simulink model "external_memory_test"  (R2020b)
settings: Solver=FixedStepDiscrete  StartTime=0.0  StopTime=80  RelTol=1e-3
InitFcn:
  | Feature_Width = 64;
  | Feature_Height = 64;
  | Weight_Width = 3;
  | Weight_Height = 3;
  | external_memory_test_init;
values from neighbouring files (symbols this model uses):
  Burst_Length = Feature_Weight_Length    [external_memory_test_init.m]
  byPass = 1    [external_memory_test_init.m]
  Conv_Padding = 0    [external_memory_test_init.m]
  Conv_Stride = 1    [external_memory_test_init.m]
  DDR_Depth = Weight_Length + Feature_Length + outFeature_Length    [external_memory_test_init.m]
  ddrInitData = single((rand(1,DDR_Depth)))    [external_memory_test_init.m]
  Duty_Cycle = 0.5    [external_memory_test_init.m]
  Feature_Area = Feature_Width * Feature_Height    [external_memory_test_init.m]
  Feature_Length = Phase_In * Feature_Area    [external_memory_test_init.m]
  inChannel = 3    [external_memory_test_init.m]
  outChannel = 2    [external_memory_test_init.m]
  outFeature_Length = outFeature_Width * outFeature_Height * Phase_Out    [external_memory_test_init.m]
  Pool_Stride = 2    [external_memory_test_init.m]
  Pool_Width = 2    [external_memory_test_init.m]
  Tc = 1    [external_memory_test_init.m]
  Ti = 1    [external_memory_test_init.m]
  To = 1    [external_memory_test_init.m]
  Tr = 1    [external_memory_test_init.m]
  Weight_Length = Phase_In * Weight_Area * Phase_Out    [external_memory_test_init.m]
undefined symbols (not defined in the file or in its folder): Conv_Step, Pool_Step, sigbuilder_block
libraries: hdlsllib x85, simulink x44, visionhdlutilities x16
(part 5 of 6)

== system external_memory_test/DUT/2DConvPE V1.3/Address Logic/  ==
  In1 : Inport
  In2 : Inport  Port=2
  Constant1 : Constant  Value=0  OutDataTypeStr=uint32
  Constant2 : Constant  Value=0  OutDataTypeStr=uint32
  Logical Operator3 : Logic  Operator=NOT  AllPortsSameDT=off  OutDataTypeStr=boolean
  Switch : Switch  Criteria=u2 ~= 0
  Switch1 : Switch  Criteria=u2 ~= 0
  addr_bit_sel1 : hdlsllib/Logic and Bit Operations/Bit Slice  lidx=12  ridx=0
  addr_bit_sel2 : hdlsllib/Logic and Bit Operations/Bit Slice  lidx=12  ridx=0
  W : Outport
  R : Outport  Port=2
  wires:
  In2/1 -> Switch/2, Logical Operator3/1
  Constant1/1 -> Switch/1
  Switch1/1 -> addr_bit_sel1/1
  In1/1 -> Switch1/3, Switch/3
  Logical Operator3/1 -> Switch1/2
  Constant2/1 -> Switch1/1
  Switch/1 -> addr_bit_sel2/1
  addr_bit_sel1/1 -> W/1  "vec_wr_addr"
  addr_bit_sel2/1 -> R/1  "vec_wr_addr"

== system external_memory_test/DUT/2DConvPE V1.3/LIne Buffer/Line Buffer ==
  Stream_In : Inport
  Stream_Valid : Inport  Port=2
  Feature_Area : Inport  Port=3
  Feature_Width : Inport  Port=4
  CtrlGen : Subsystem
  Line Buffer : visionhdlutilities/Line Buffer  NeighborhoodSize=[3 1]  PaddingMethod=Constant  PaddingValue=0  LineBufferSize=128  SimulateUsing=Code generation
      settings: SourceProductBaseCode=VT
  pixel : Outport
  ctrl : Outport  Port=2
  shftEnable : Outport  Port=3
  wires:
  Feature_Area/1 -> CtrlGen/3(Feature_Area)
  Line Buffer/2 -> ctrl/1
  CtrlGen/1(StreamOut) -> Line Buffer/1
  Feature_Width/1 -> CtrlGen/4(Feature_Width)
  Stream_In/1 -> CtrlGen/1(Stream_In)
  CtrlGen/2(Ctrl) -> Line Buffer/2
  Stream_Valid/1 -> CtrlGen/2(Stream_Valid)
  Line Buffer/3 -> shftEnable/1
  Line Buffer/1 -> pixel/1

== system external_memory_test/DUT/2DConvPE V1.3/LIne Buffer/OutValidGen ==
  In1 : Inport
  Weight_Width : Inport  Port=2
  Feature_Height : Inport  Port=3
  Compare To Constant : simulink/Logic and Bit Operations/Compare To Constant  relop=>  const=0  OutDataTypeStr=boolean
  Constant : Constant  OutDataTypeStr=uint32  SampleTime=-1
  Delay2 : Delay  DelayLength=1
  Logical Operator1 : Logic  Operator=NOT  AllPortsSameDT=off  OutDataTypeStr=boolean
  Logical Operator2 : Logic  Operator=OR  AllPortsSameDT=off  OutDataTypeStr=boolean
  Logical Operator3 : Logic  Inputs=4  AllPortsSameDT=off  OutDataTypeStr=boolean
  Logical Operator4 : Logic  Operator=NOT  AllPortsSameDT=off  OutDataTypeStr=boolean
  Logical Operator5 : Logic  Operator=OR  AllPortsSameDT=off  OutDataTypeStr=boolean
  Logical Operator6 : Logic  Operator=NOT  Inputs=3  AllPortsSameDT=off  OutDataTypeStr=boolean
  Minus1 : Sum  Inputs=+--
  Minus2 : Sum  Inputs=+-
  NumRow_Counter : hdlsllib/Sources/HDL Counter  CountType=Free running  CountInit=0  CountStep=1  CountMax=2^15  CountFromType=Initial value  CountFrom=0  CountResetPort=on  CountLoadPort=off  CountEnbPort=on  CountDirPort=off  CountDataType=Unsigned  CountWordLen=32  CountFracLen=0  CountSampTime=1
  Pixel Control Bus Selector : BusSelector  OutputSignals=hStart,hEnd,vStart,vEnd,valid
  Relational Operator1 : RelationalOperator  Operator=<  OutDataTypeStr=boolean  RndMeth=Nearest
  Relational Operator2 : RelationalOperator  Operator=<=  OutDataTypeStr=boolean  RndMeth=Nearest
  Row_Counter : hdlsllib/Sources/HDL Counter  CountType=Free running  CountInit=0  CountStep=1  CountMax=2^15  CountFromType=Initial value  CountFrom=0  CountResetPort=on  CountLoadPort=off  CountEnbPort=on  CountDirPort=off  CountDataType=Unsigned  CountWordLen=32  CountFracLen=0  CountSampTime=1
  Terminator1 : Terminator
  valid : Outport
  wires:
  Compare To Constant/1 -> Logical Operator3/2
  NumRow_Counter/1 -> Relational Operator2/2, Compare To Constant/1
  Pixel Control Bus Selector/1 -> NumRow_Counter/2, Logical Operator2/1  "<hStart>"
  Minus2/1 -> Relational Operator2/1
  Relational Operator1/1 -> Logical Operator4/1
  Logical Operator1/1 -> Logical Operator2/2
  Pixel Control Bus Selector/3 -> Logical Operator5/1  "<vStart>"
  Feature_Height/1 -> Minus2/1
  Minus1/1 -> Relational Operator1/2
  Row_Counter/1 -> Relational Operator1/1
  Pixel Control Bus Selector/5 -> Logical Operator1/1, Row_Counter/2, Logical Operator3/3  "<valid>"
  Weight_Width/1 -> Minus1/1
  Pixel Control Bus Selector/2 -> Terminator1/1  "<hEnd>"
  Delay2/1 -> Pixel Control Bus Selector/1
  Constant/1 -> Minus1/3, Minus1/2, Minus2/2
  Logical Operator6/1 -> Logical Operator3/1
  Logical Operator5/1 -> NumRow_Counter/1
  Pixel Control Bus Selector/4 -> Logical Operator5/2  "<vEnd>"
  Relational Operator2/1 -> Logical Operator6/1
  Logical Operator2/1 -> Row_Counter/1
  Logical Operator4/1 -> Logical Operator3/4
  Logical Operator3/1 -> valid/1
  In1/1 -> Delay2/1

== system external_memory_test/DUT/2DConvPE V1.3/MaxPooling/Comparator ==
  In1 : Inport
  In2 : Inport  Port=2
  In3 : Inport  Port=3
  In4 : Inport  Port=4
  Valid : Inport  Port=5
  Delay{,1..4} (5 alike) : Delay  DelayLength=1
  Relational Operator : RelationalOperator  Operator=>  OutDataTypeStr=boolean  RndMeth=Nearest
  Relational Operator1 : RelationalOperator  Operator=>  OutDataTypeStr=boolean  RndMeth=Nearest
  Relational Operator2 : RelationalOperator  Operator=>  OutDataTypeStr=boolean  RndMeth=Nearest
  Switch : Switch  Criteria=u2 > Threshold
  Switch1 : Switch  Criteria=u2 > Threshold
  Switch2 : Switch  Criteria=u2 > Threshold
  Out1 : Outport
  outvalid : Outport  Port=2
  wires:
  Switch1/1 -> Relational Operator2/2, Switch2/3
  Switch/1 -> Switch2/1, Relational Operator2/1
  Delay/1 -> Switch/1, Relational Operator/1
  Relational Operator/1 -> Switch/2
  Relational Operator1/1 -> Switch1/2
  In2/1 -> Delay1/1
  In3/1 -> Delay2/1
  Relational Operator2/1 -> Switch2/2
  In4/1 -> Delay3/1
  Switch2/1 -> Out1/1
  Valid/1 -> Delay4/1
  Delay1/1 -> Relational Operator/2, Switch/3
  Delay2/1 -> Switch1/1, Relational Operator1/1
  In1/1 -> Delay/1
  Delay3/1 -> Relational Operator1/2, Switch1/3
  Delay4/1 -> outvalid/1

== system external_memory_test/DUT/2DConvPE V1.3/MaxPooling/Line Buffer1 ==
  Stream_In : Inport
  Stream_Valid : Inport  Port=2
  Feature_Area : Inport  Port=3
  Feature_Width : Inport  Port=4
  CtrlGen : Subsystem
  Line Buffer : visionhdlutilities/Line Buffer  NeighborhoodSize=[2 1]  PaddingMethod=Constant  PaddingValue=0  LineBufferSize=128  SimulateUsing=Code generation
      settings: SourceProductBaseCode=VT
  pixel : Outport
  ctrl : Outport  Port=2
  shftEnable : Outport  Port=3
  wires:
  Feature_Area/1 -> CtrlGen/3(Feature_Area)
  Line Buffer/2 -> ctrl/1
  CtrlGen/1(StreamOut) -> Line Buffer/1
  Feature_Width/1 -> CtrlGen/4(Feature_Width)
  Stream_In/1 -> CtrlGen/1(Stream_In)
  CtrlGen/2(Ctrl) -> Line Buffer/2
  Stream_Valid/1 -> CtrlGen/2(Stream_Valid)
  Line Buffer/3 -> shftEnable/1
  Line Buffer/1 -> pixel/1

== system external_memory_test/DUT/2DConvPE V1.3/MaxPooling/OutValidGen ==
  ctrl : Inport
  Window_Width : Inport  Port=2
  Feature_Height : Inport  Port=3
  Compare To Constant : simulink/Logic and Bit Operations/Compare To Constant  Commented=on  relop=>  const=0  OutDataTypeStr=boolean
  Constant : Constant  OutDataTypeStr=uint32  SampleTime=-1
  Delay36 : Delay  DelayLength=1
  Logical Operator1 : Logic  Operator=NOT  AllPortsSameDT=off  OutDataTypeStr=boolean
  Logical Operator3 : Logic  Inputs=3  AllPortsSameDT=off  OutDataTypeStr=boolean
  Logical Operator4 : Logic  Operator=NOT  AllPortsSameDT=off  OutDataTypeStr=boolean
  Logical Operator5 : Logic  Operator=OR  AllPortsSameDT=off  OutDataTypeStr=boolean
  Logical Operator6 : Logic  Operator=NOT  Inputs=3  AllPortsSameDT=off  OutDataTypeStr=boolean
  Minus1 : Sum  Inputs=+-
  Minus2 : Sum  Inputs=+-
  NumRow_Counter : hdlsllib/Sources/HDL Counter  CountType=Free running  CountInit=0  CountStep=1  CountMax=2^15  CountFromType=Initial value  CountFrom=0  CountResetPort=on  CountLoadPort=off  CountEnbPort=on  CountDirPort=off  CountDataType=Unsigned  CountWordLen=32  CountFracLen=0  CountSampTime=1
  Pixel Control Bus Selector : BusSelector  OutputSignals=hStart,hEnd,vStart,vEnd,valid
  Relational Operator1 : RelationalOperator  Operator=<  OutDataTypeStr=boolean  RndMeth=Nearest
  Relational Operator2 : RelationalOperator  Operator=<=  OutDataTypeStr=boolean  RndMeth=Nearest
  Row_Counter : hdlsllib/Sources/HDL Counter  CountType=Free running  CountInit=0  CountStep=1  CountMax=2^15  CountFromType=Initial value  CountFrom=0  CountResetPort=on  CountLoadPort=off  CountEnbPort=on  CountDirPort=off  CountDataType=Unsigned  CountWordLen=32  CountFracLen=0  CountSampTime=1
  Terminator1 : Terminator
  Out1 : Outport
  wires:
  NumRow_Counter/1 -> Relational Operator2/2, Compare To Constant/1
  Pixel Control Bus Selector/1 -> NumRow_Counter/2  "<hStart>"
  Minus2/1 -> Relational Operator2/1
  Relational Operator1/1 -> Logical Operator4/1
  Pixel Control Bus Selector/3 -> Logical Operator5/1  "<vStart>"
  Feature_Height/1 -> Minus2/1
  Minus1/1 -> Relational Operator1/2
  Row_Counter/1 -> Relational Operator1/1
  Pixel Control Bus Selector/5 -> Row_Counter/2, Logical Operator1/1, Logical Operator3/2  "<valid>"
  Window_Width/1 -> Minus1/1
  Pixel Control Bus Selector/2 -> Terminator1/1  "<hEnd>"
  Delay36/1 -> Pixel Control Bus Selector/1
  Constant/1 -> Minus1/2, Minus2/2
  Logical Operator6/1 -> Logical Operator3/1
  Logical Operator5/1 -> NumRow_Counter/1
  Pixel Control Bus Selector/4 -> Logical Operator5/2  "<vEnd>"
  Relational Operator2/1 -> Logical Operator6/1
  Logical Operator1/1 -> Row_Counter/1
  Logical Operator4/1 -> Logical Operator3/3
  Logical Operator3/1 -> Out1/1
  ctrl/1 -> Delay36/1

== system external_memory_test/DUT/2DConvPE V1.3/MaxPooling/window Selector ==
  pixel : Inport
  valid : Inport  Port=2
  step : Inport  Port=3
  Add : Sum  Inputs=+-
  Compare To Zero : simulink/Logic and Bit Operations/Compare To Zero  relop===  OutDataTypeStr=boolean
  Constant : Constant  OutDataTypeStr=uint32
  Delay : Delay
  Delay1 : Delay  DelayLength=1
  Delay36 : Delay  DelayLength=1
  Logical Operator : Logic  Operator=NOT  AllPortsSameDT=off  OutDataTypeStr=boolean
  Logical Operator1 : Logic  Operator=OR  AllPortsSameDT=off  OutDataTypeStr=boolean
  Logical Operator2 : Logic  AllPortsSameDT=off  OutDataTypeStr=boolean
  Relational Operator : RelationalOperator  OutDataTypeStr=boolean  RndMeth=Nearest
  Selector1 : Selector  InputPortWidth=2  IndexOptions=Index vector (dialog)  Indices=[1]  OutputSizes=1
  Selector2 : Selector  InputPortWidth=2  IndexOptions=Index vector (dialog)  Indices=[2]  OutputSizes=1
  Selector3 : Selector  InputPortWidth=2  IndexOptions=Index vector (dialog)  Indices=[1]  OutputSizes=1
  Selector4 : Selector  InputPortWidth=2  IndexOptions=Index vector (dialog)  Indices=[2]  OutputSizes=1
  Step Counter : hdlsllib/Sources/HDL Counter  CountType=Free running  CountInit=0  CountStep=1  CountMax=2^15  CountFromType=Initial value  CountFrom=0  CountResetPort=on  CountLoadPort=off  CountEnbPort=on  CountDirPort=off  CountDataType=Unsigned  CountWordLen=32  CountFracLen=0  CountSampTime=1
  Out1 : Outport
  Out2 : Outport  Port=2
  Out3 : Outport  Port=3
  Out4 : Outport  Port=4
  Valid : Outport  Port=5
  wires:
  Selector2/1 -> Out2/1
  Delay/1 -> Selector4/1, Selector3/1
  Selector3/1 -> Out3/1
  Selector1/1 -> Out1/1
  Selector4/1 -> Out4/1
  pixel/1 -> Delay36/1, Delay/1
  Step Counter/1 -> Compare To Zero/1, Relational Operator/1
  Delay1/1 -> Logical Operator2/2, Step Counter/2, Logical Operator/1
  Logical Operator/1 -> Logical Operator1/2
  step/1 -> Add/1
  Constant/1 -> Add/2
  Add/1 -> Relational Operator/2
  Relational Operator/1 -> Logical Operator1/1
  Logical Operator1/1 -> Step Counter/1
  Compare To Zero/1 -> Logical Operator2/1
  Logical Operator2/1 -> Valid/1
  Delay36/1 -> Selector2/1, Selector1/1
  valid/1 -> Delay1/1

== system external_memory_test/DUT/Input Buffer/OutAddressLogic/FeatureAddressOut ==
  note: FeatureDelay May Correlated to Line Buffer Window
  Feature_Length : Inport
  Out_Enable : Inport  Port=2
  Feature_Width : Inport  Port=3
  outChannel : Inport  Port=4
  Feature_Height : Inport  Port=5
  " FeatureDelay" : Constant  OutDataTypeStr=uint32  SampleTime=-1
  Add{1..2,4,6} (4 alike) : Sum  Inputs=+-
  Add3 : Sum
  Add5 : Sum
  Constant1 : Constant  OutDataTypeStr=uint32  SampleTime=-1
  Feature_Length_Counter : hdlsllib/Sources/HDL Counter  CountType=Free running  CountInit=0  CountStep=1  CountMax=2^15  CountFromType=Initial value  CountFrom=0  CountResetPort=on  CountLoadPort=off  CountEnbPort=on  CountDirPort=off  CountDataType=Unsigned  CountWordLen=32  CountFracLen=0  CountSampTime=1
  Iteration_Counter : hdlsllib/Sources/HDL Counter  CountType=Free running  CountInit=0  CountStep=1  CountMax=2^15  CountFromType=Initial value  CountFrom=0  CountResetPort=on  CountLoadPort=off  CountEnbPort=on  CountDirPort=off  CountDataType=Unsigned  CountWordLen=32  CountFracLen=0  CountSampTime=1
  Logical Operator{,2,4..5} (4 alike) : Logic  Operator=NOT  AllPortsSameDT=off  OutDataTypeStr=boolean
  Logical Operator1 : Logic  Inputs=3  AllPortsSameDT=off  OutDataTypeStr=boolean
  Logical Operator3 : Logic  AllPortsSameDT=off  OutDataTypeStr=boolean
  Logical Operator6 : Logic  Operator=OR  AllPortsSameDT=off  OutDataTypeStr=boolean
  Relational Operator{1..6} (6 alike) : RelationalOperator  Operator=>  OutDataTypeStr=boolean  RndMeth=Simplest
  Row+Delay_Counter : hdlsllib/Sources/HDL Counter  CountType=Free running  CountInit=0  CountStep=1  CountMax=2^15  CountFromType=Initial value  CountFrom=0  CountResetPort=on  CountLoadPort=off  CountEnbPort=on  CountDirPort=off  CountDataType=Unsigned  CountWordLen=32  CountFracLen=0  CountSampTime=1
  RowDelay : Constant  OutDataTypeStr=uint32  SampleTime=-1
  Row_Counter : hdlsllib/Sources/HDL Counter  CountType=Free running  CountInit=0  CountStep=1  CountMax=2^15  CountFromType=Initial value  CountFrom=0  CountResetPort=on  CountLoadPort=off  CountEnbPort=on  CountDirPort=off  CountDataType=Unsigned  CountWordLen=32  CountFracLen=0  CountSampTime=1
  count : Outport
  Out2 : Outport  Port=2
  PhaseOut_Count : Outport  Port=3
  wires:
  RowDelay/1 -> Add3/1
  Out_Enable/1 -> Logical Operator3/2, Logical Operator4/1
  Row+Delay_Counter/1 -> Relational Operator2/1, Relational Operator1/1
  Add4/1 -> Relational Operator4/2
  Constant1/1 -> Add6/2, Add2/2, Add4/2, Add1/2
  Relational Operator3/1 -> Feature_Length_Counter/1, Iteration_Counter/2
  Logical Operator1/1 -> Out2/1, Feature_Length_Counter/2
  Iteration_Counter/1 -> Relational Operator4/1, PhaseOut_Count/1
  Relational Operator4/1 -> Logical Operator2/1
  Relational Operator2/1 -> Logical Operator/1
  Logical Operator3/1 -> Row+Delay_Counter/2, Logical Operator1/1
  Add1/1 -> Relational Operator3/2
  Add3/1 -> Relational Operator1/2
  Relational Operator1/1 -> Logical Operator6/1, Row_Counter/2
  Logical Operator4/1 -> Iteration_Counter/1
  Add2/1 -> Relational Operator2/2, Add3/2
  Logical Operator/1 -> Logical Operator1/2
  Feature_Length_Counter/1 -> count/1, Relational Operator3/1
  Logical Operator2/1 -> Logical Operator3/1
  Feature_Width/1 -> Add2/1
  Feature_Length/1 -> Add1/1
  outChannel/1 -> Add4/1
  Add5/1 -> Relational Operator5/2
  Row_Counter/1 -> Relational Operator5/1, Relational Operator6/1
  Feature_Height/1 -> Add5/2, Add6/1
  " FeatureDelay"/1 -> Add5/1
  Relational Operator5/1 -> Row_Counter/1, Logical Operator6/2
  Add6/1 -> Relational Operator6/2
  Relational Operator6/1 -> Logical Operator5/1
  Logical Operator5/1 -> Logical Operator1/3
  Logical Operator6/1 -> Row+Delay_Counter/1

== system external_memory_test/DUT/Input Buffer/OutAddressLogic/Subsystem ==
  In1 : Inport
  Feature_Area : Inport  Port=2
  Weight_Length : Inport  Port=3
  Weight_Area : Inport  Port=4
  Add1 : Sum  Inputs=+-
  Add2 : Sum  Inputs=+-
  Add3 : Sum  Inputs=+-
  Constant1 : Constant  OutDataTypeStr=uint32  SampleTime=-1
  Feature_Area_Count : hdlsllib/Sources/HDL Counter  CountType=Free running  CountInit=0  CountStep=1  CountMax=2^15  CountFromType=Initial value  CountFrom=0  CountResetPort=on  CountLoadPort=off  CountEnbPort=on  CountDirPort=off  CountDataType=Unsigned  CountWordLen=32  CountFracLen=0  CountSampTime=1
  Logical Operator1 : Logic  Operator=NOT  AllPortsSameDT=off  OutDataTypeStr=boolean
  Logical Operator2 : Logic  Operator=NOT  AllPortsSameDT=off  OutDataTypeStr=boolean
  Logical Operator3 : Logic  AllPortsSameDT=off  OutDataTypeStr=boolean
  Relational Operator2 : RelationalOperator  Operator=>  OutDataTypeStr=boolean  RndMeth=Simplest
  Relational Operator3 : RelationalOperator  Operator=>  OutDataTypeStr=boolean  RndMeth=Simplest
  Relational Operator4 : RelationalOperator  Operator=<=  OutDataTypeStr=boolean  RndMeth=Simplest
  Weight_Length_Count : hdlsllib/Sources/HDL Counter  CountType=Free running  CountInit=0  CountStep=1  CountMax=2^15  CountFromType=Initial value  CountFrom=0  CountResetPort=on  CountLoadPort=off  CountEnbPort=on  CountDirPort=off  CountDataType=Unsigned  CountWordLen=32  CountFracLen=0  CountSampTime=1
  weight_ram_rd_addr : Outport
  valid : Outport  Port=2
  wires:
  Relational Operator4/1 -> Logical Operator3/2
  Weight_Length/1 -> Add1/1
  Feature_Area/1 -> Add2/1
  Constant1/1 -> Add3/2, Add1/2, Add2/2
  Weight_Length_Count/1 -> weight_ram_rd_addr/1, Relational Operator2/2
  Relational Operator2/1 -> Logical Operator1/1
  Logical Operator3/1 -> valid/1, Weight_Length_Count/2
  Feature_Area_Count/1 -> Relational Operator4/1, Relational Operator3/2
  In1/1 -> Logical Operator3/1, Feature_Area_Count/2
  Add2/1 -> Relational Operator3/1
  Add3/1 -> Relational Operator4/2
  Add1/1 -> Relational Operator2/1
  Logical Operator2/1 -> Feature_Area_Count/1
  Relational Operator3/1 -> Logical Operator2/1
  Logical Operator1/1 -> Weight_Length_Count/1
  Weight_Area/1 -> Add3/1

== system external_memory_test/DUT/Input Buffer/Subsystem1/Subsystem ==
  In1 : Inport
  Bus Selector : BusSelector  OutputSignals=signal1,signal2,signal3,signal4,signal5,signal6,signal7,signal8,signal9,signal10,signal11,signal12,signal13,signal14,signal15
  Weight_Length : Outport
  Weight_Area : Outport  Port=2
  Weight_Width : Outport  Port=3
  Weight_Height : Outport  Port=4
  Feature_Length : Outport  Port=5
  Feature_Area : Outport  Port=6
  Feature_Width : Outport  Port=7
  Feature_Height : Outport  Port=8
  outFeature_Length : Outport  Port=9
  outFeature_Area : Outport  Port=10
  outFeature_Width : Outport  Port=11
  outFeature_Height : Outport  Port=12
  Conv_Step : Outport  Port=13
  inChannel : Outport  Port=14
  outChannel : Outport  Port=15
  wires:
  In1/1 -> Bus Selector/1
  Bus Selector/1 -> Weight_Length/1  "<signal1>"
  Bus Selector/2 -> Weight_Area/1  "<signal2>"
  Bus Selector/3 -> Weight_Width/1  "<signal3>"
  Bus Selector/4 -> Weight_Height/1  "<signal4>"
  Bus Selector/5 -> Feature_Length/1  "<signal5>"
  Bus Selector/6 -> Feature_Area/1  "<signal6>"
  Bus Selector/7 -> Feature_Width/1  "<signal7>"
  Bus Selector/8 -> Feature_Height/1  "<signal8>"
  Bus Selector/9 -> outFeature_Length/1  "<signal9>"
  Bus Selector/10 -> outFeature_Area/1  "<signal10>"
  Bus Selector/11 -> outFeature_Width/1  "<signal11>"
  Bus Selector/12 -> outFeature_Height/1  "<signal12>"
  Bus Selector/13 -> Conv_Step/1  "<signal13>"
  Bus Selector/14 -> inChannel/1  "<signal14>"
  Bus Selector/15 -> outChannel/1  "<signal15>"

== system external_memory_test/DDR/wrLogic/Wr_control/AckGen/edgeDet ==
  ackIn : Inport
  " ackIn==1" : simulink/Logic and Bit Operations/Compare To Constant  relop===  const=1  OutDataTypeStr=boolean
  ackIn Posedge Detect : Logic  IconShape=distinctive  AllPortsSameDT=off  OutDataTypeStr=boolean
  ackIn_d1 : Delay  DelayLength=1
  ackIn_d1==0 : simulink/Logic and Bit Operations/Compare To Constant  relop===  const=0  OutDataTypeStr=boolean
  ackOut : Outport  VectorParamsAs1DForOutWhenUnconnected=off
  wires:
  " ackIn==1"/1 -> ackIn Posedge Detect/2
  ackIn_d1==0/1 -> ackIn Posedge Detect/1
  ackIn Posedge Detect/1 -> ackOut/1
  ackIn_d1/1 -> ackIn_d1==0/1
  ackIn/1 -> " ackIn==1"/1, ackIn_d1/1

== system external_memory_test/DUT/2DConvPE V1.0/LIne Buffer/Line Buffer/CtrlGen ==
  note: valid
  note: vEnd
  note: vStart
  note: hEnd
  note: hstart
  Stream_In : Inport
  Stream_Valid : Inport  Port=2
  Feature_Area : Inport  Port=3
  Feature_Width : Inport  Port=4
  Compare To Zero : simulink/Logic and Bit Operations/Compare To Zero  relop===  OutDataTypeStr=boolean
  Compare To Zero1 : simulink/Logic and Bit Operations/Compare To Zero  relop===  OutDataTypeStr=boolean
  Constant : Constant  OutDataTypeStr=uint32  SampleTime=-1
  Constant1 : Constant  OutDataTypeStr=uint32  SampleTime=-1
  Delay3 : Delay  DelayLength=1
  Delay35 : Delay  DelayLength=1
  Feature Area Counter : hdlsllib/Sources/HDL Counter  CountType=Free running  CountInit=0  CountStep=1  CountMax=2^15  CountFromType=Initial value  CountFrom=0  CountResetPort=on  CountLoadPort=off  CountEnbPort=on  CountDirPort=off  CountDataType=Unsigned  CountWordLen=32  CountFracLen=0  CountSampTime=1
  Feature Row Counter : hdlsllib/Sources/HDL Counter  CountType=Free running  CountInit=0  CountStep=1  CountMax=2^15  CountFromType=Initial value  CountFrom=0  CountResetPort=on  CountLoadPort=off  CountEnbPort=on  CountDirPort=off  CountDataType=Unsigned  CountWordLen=32  CountFracLen=0  CountSampTime=1
  Logical Operator : Logic  Operator=OR  AllPortsSameDT=off  OutDataTypeStr=boolean
  Logical Operator{1..3,5} (4 alike) : Logic  AllPortsSameDT=off  OutDataTypeStr=boolean
  Minus1 : Sum  Inputs=+-
  Minus2 : Sum  Inputs=+-
  Pixel Control Bus Creator : visionhdlutilities/Pixel Control Bus Creator
      settings: SourceProductBaseCode=VT
  Relational Operator1 : RelationalOperator  Operator===  OutDataTypeStr=boolean  RndMeth=Nearest
  Relational Operator2 : RelationalOperator  Operator===  OutDataTypeStr=boolean  RndMeth=Nearest
  Relational Operator3 : RelationalOperator  Operator===  OutDataTypeStr=boolean  RndMeth=Nearest
  StreamOut : Outport
  Ctrl : Outport  Port=2
  wires:
  Minus2/1 -> Relational Operator3/2, Relational Operator2/2
  Feature Row Counter/1 -> Relational Operator2/1, Relational Operator3/1, Compare To Zero/1
  Relational Operator2/1 -> Feature Row Counter/1
  Compare To Zero/1 -> Logical Operator/2
  Relational Operator3/1 -> Logical Operator2/1
  Feature_Area/1 -> Minus1/1
  Constant/1 -> Minus1/2
  Logical Operator/1 -> Logical Operator1/1
  Constant1/1 -> Minus2/2
  Feature_Width/1 -> Minus2/1
  Pixel Control Bus Creator/1 -> Ctrl/1
  Delay3/1 -> Feature Area Counter/2, Feature Row Counter/2, Logical Operator5/2, Logical Operator2/2, Logical Operator1/2, Logical Operator3/2, Pixel Control Bus Creator/5
  Stream_In/1 -> Delay35/1
  Logical Operator1/1 -> Pixel Control Bus Creator/1
  Logical Operator2/1 -> Pixel Control Bus Creator/2
  Logical Operator3/1 -> Pixel Control Bus Creator/4
  Logical Operator5/1 -> Pixel Control Bus Creator/3
  Feature Area Counter/1 -> Compare To Zero1/1, Relational Operator1/1
  Minus1/1 -> Relational Operator1/2
  Relational Operator1/1 -> Feature Area Counter/1, Logical Operator3/1
  Compare To Zero1/1 -> Logical Operator/1, Logical Operator5/1
  Delay35/1 -> StreamOut/1
  Stream_Valid/1 -> Delay3/1

== system external_memory_test/DUT/2DConvPE V1.0/MaxPooling/Line Buffer1/CtrlGen ==
  note: valid
  note: vEnd
  note: vStart
  note: hEnd
  note: hstart
  Stream_In : Inport
  Stream_Valid : Inport  Port=2
  Feature_Area : Inport  Port=3
  Feature_Width : Inport  Port=4
  Compare To Zero : simulink/Logic and Bit Operations/Compare To Zero  relop===  OutDataTypeStr=boolean
  Compare To Zero1 : simulink/Logic and Bit Operations/Compare To Zero  relop===  OutDataTypeStr=boolean
  Constant : Constant  OutDataTypeStr=uint32  SampleTime=-1
  Constant1 : Constant  OutDataTypeStr=uint32  SampleTime=-1
  Delay1 : Delay  DelayLength=1
  Delay36 : Delay  DelayLength=1
  Feature Area Counter : hdlsllib/Sources/HDL Counter  CountType=Free running  CountInit=0  CountStep=1  CountMax=2^15  CountFromType=Initial value  CountFrom=0  CountResetPort=on  CountLoadPort=off  CountEnbPort=on  CountDirPort=off  CountDataType=Unsigned  CountWordLen=32  CountFracLen=0  CountSampTime=1
  Feature Row Counter : hdlsllib/Sources/HDL Counter  CountType=Free running  CountInit=0  CountStep=1  CountMax=2^15  CountFromType=Initial value  CountFrom=0  CountResetPort=on  CountLoadPort=off  CountEnbPort=on  CountDirPort=off  CountDataType=Unsigned  CountWordLen=32  CountFracLen=0  CountSampTime=1
  Logical Operator : Logic  Operator=OR  AllPortsSameDT=off  OutDataTypeStr=boolean
  Logical Operator{1..3,5} (4 alike) : Logic  AllPortsSameDT=off  OutDataTypeStr=boolean
  Minus1 : Sum  Inputs=+-
  Minus2 : Sum  Inputs=+-
  Pixel Control Bus Creator : visionhdlutilities/Pixel Control Bus Creator
      settings: SourceProductBaseCode=VT
  Relational Operator1 : RelationalOperator  Operator===  OutDataTypeStr=boolean  RndMeth=Nearest
  Relational Operator2 : RelationalOperator  Operator===  OutDataTypeStr=boolean  RndMeth=Nearest
  Relational Operator3 : RelationalOperator  Operator===  OutDataTypeStr=boolean  RndMeth=Nearest
  StreamOut : Outport
  Ctrl : Outport  Port=2
  wires:
  Minus2/1 -> Relational Operator3/2, Relational Operator2/2
  Feature Row Counter/1 -> Relational Operator2/1, Relational Operator3/1, Compare To Zero/1
  Relational Operator2/1 -> Feature Row Counter/1
  Compare To Zero/1 -> Logical Operator/2
  Relational Operator3/1 -> Logical Operator2/1
  Feature_Area/1 -> Minus1/1
  Constant/1 -> Minus1/2
  Logical Operator/1 -> Logical Operator1/1
  Constant1/1 -> Minus2/2
  Feature_Width/1 -> Minus2/1
  Pixel Control Bus Creator/1 -> Ctrl/1
  Delay1/1 -> Feature Area Counter/2, Feature Row Counter/2, Logical Operator5/2, Logical Operator2/2, Logical Operator1/2, Logical Operator3/2, Pixel Control Bus Creator/5
  Delay36/1 -> StreamOut/1
  Logical Operator1/1 -> Pixel Control Bus Creator/1
  Logical Operator2/1 -> Pixel Control Bus Creator/2
  Logical Operator3/1 -> Pixel Control Bus Creator/4
  Logical Operator5/1 -> Pixel Control Bus Creator/3
  Feature Area Counter/1 -> Compare To Zero1/1, Relational Operator1/1
  Minus1/1 -> Relational Operator1/2
  Relational Operator1/1 -> Feature Area Counter/1, Logical Operator3/1
  Compare To Zero1/1 -> Logical Operator/1, Logical Operator5/1
  Stream_In/1 -> Delay36/1
  Stream_Valid/1 -> Delay1/1

== system external_memory_test/DUT/2DConvPE V1.1/LIne Buffer/Line Buffer/CtrlGen ==
  note: valid
  note: vEnd
  note: vStart
  note: hEnd
  note: hstart
  Stream_In : Inport
  Stream_Valid : Inport  Port=2
  Feature_Area : Inport  Port=3
  Feature_Width : Inport  Port=4
  Compare To Zero : simulink/Logic and Bit Operations/Compare To Zero  relop===  OutDataTypeStr=boolean
  Compare To Zero1 : simulink/Logic and Bit Operations/Compare To Zero  relop===  OutDataTypeStr=boolean
  Constant : Constant  OutDataTypeStr=uint32  SampleTime=-1
  Constant1 : Constant  OutDataTypeStr=uint32  SampleTime=-1
  Delay3 : Delay  DelayLength=1
  Delay35 : Delay  DelayLength=1
  Feature Area Counter : hdlsllib/Sources/HDL Counter  CountType=Free running  CountInit=0  CountStep=1  CountMax=2^15  CountFromType=Initial value  CountFrom=0  CountResetPort=on  CountLoadPort=off  CountEnbPort=on  CountDirPort=off  CountDataType=Unsigned  CountWordLen=32  CountFracLen=0  CountSampTime=1
  Feature Row Counter : hdlsllib/Sources/HDL Counter  CountType=Free running  CountInit=0  CountStep=1  CountMax=2^15  CountFromType=Initial value  CountFrom=0  CountResetPort=on  CountLoadPort=off  CountEnbPort=on  CountDirPort=off  CountDataType=Unsigned  CountWordLen=32  CountFracLen=0  CountSampTime=1
  Logical Operator : Logic  Operator=OR  AllPortsSameDT=off  OutDataTypeStr=boolean
  Logical Operator{1..3,5} (4 alike) : Logic  AllPortsSameDT=off  OutDataTypeStr=boolean
  Minus1 : Sum  Inputs=+-
  Minus2 : Sum  Inputs=+-
  Pixel Control Bus Creator : visionhdlutilities/Pixel Control Bus Creator
      settings: SourceProductBaseCode=VT
  Relational Operator1 : RelationalOperator  Operator===  OutDataTypeStr=boolean  RndMeth=Nearest
  Relational Operator2 : RelationalOperator  Operator===  OutDataTypeStr=boolean  RndMeth=Nearest
  Relational Operator3 : RelationalOperator  Operator===  OutDataTypeStr=boolean  RndMeth=Nearest
  StreamOut : Outport
  Ctrl : Outport  Port=2
  wires:
  Minus2/1 -> Relational Operator3/2, Relational Operator2/2
  Feature Row Counter/1 -> Relational Operator2/1, Relational Operator3/1, Compare To Zero/1
  Relational Operator2/1 -> Feature Row Counter/1
  Compare To Zero/1 -> Logical Operator/2
  Relational Operator3/1 -> Logical Operator2/1
  Feature_Area/1 -> Minus1/1
  Constant/1 -> Minus1/2
  Logical Operator/1 -> Logical Operator1/1
  Constant1/1 -> Minus2/2
  Feature_Width/1 -> Minus2/1
  Pixel Control Bus Creator/1 -> Ctrl/1
  Delay3/1 -> Feature Area Counter/2, Feature Row Counter/2, Logical Operator5/2, Logical Operator2/2, Logical Operator1/2, Logical Operator3/2, Pixel Control Bus Creator/5
  Stream_In/1 -> Delay35/1
  Logical Operator1/1 -> Pixel Control Bus Creator/1
  Logical Operator2/1 -> Pixel Control Bus Creator/2
  Logical Operator3/1 -> Pixel Control Bus Creator/4
  Logical Operator5/1 -> Pixel Control Bus Creator/3
  Feature Area Counter/1 -> Compare To Zero1/1, Relational Operator1/1
  Minus1/1 -> Relational Operator1/2
  Relational Operator1/1 -> Feature Area Counter/1, Logical Operator3/1
  Compare To Zero1/1 -> Logical Operator/1, Logical Operator5/1
  Delay35/1 -> StreamOut/1
  Stream_Valid/1 -> Delay3/1

== system external_memory_test/DUT/2DConvPE V1.1/MaxPooling/Line Buffer1/CtrlGen ==
  note: valid
  note: vEnd
  note: vStart
  note: hEnd
  note: hstart
  Stream_In : Inport
  Stream_Valid : Inport  Port=2
  Feature_Area : Inport  Port=3
  Feature_Width : Inport  Port=4
  Compare To Zero : simulink/Logic and Bit Operations/Compare To Zero  relop===  OutDataTypeStr=boolean
  Compare To Zero1 : simulink/Logic and Bit Operations/Compare To Zero  relop===  OutDataTypeStr=boolean
  Constant : Constant  OutDataTypeStr=uint32  SampleTime=-1
  Constant1 : Constant  OutDataTypeStr=uint32  SampleTime=-1
  Delay1 : Delay  DelayLength=1
  Delay36 : Delay  DelayLength=1
  Feature Area Counter : hdlsllib/Sources/HDL Counter  CountType=Free running  CountInit=0  CountStep=1  CountMax=2^15  CountFromType=Initial value  CountFrom=0  CountResetPort=on  CountLoadPort=off  CountEnbPort=on  CountDirPort=off  CountDataType=Unsigned  CountWordLen=32  CountFracLen=0  CountSampTime=1
  Feature Row Counter : hdlsllib/Sources/HDL Counter  CountType=Free running  CountInit=0  CountStep=1  CountMax=2^15  CountFromType=Initial value  CountFrom=0  CountResetPort=on  CountLoadPort=off  CountEnbPort=on  CountDirPort=off  CountDataType=Unsigned  CountWordLen=32  CountFracLen=0  CountSampTime=1
  Logical Operator : Logic  Operator=OR  AllPortsSameDT=off  OutDataTypeStr=boolean
  Logical Operator{1..3,5} (4 alike) : Logic  AllPortsSameDT=off  OutDataTypeStr=boolean
  Minus1 : Sum  Inputs=+-
  Minus2 : Sum  Inputs=+-
  Pixel Control Bus Creator : visionhdlutilities/Pixel Control Bus Creator
      settings: SourceProductBaseCode=VT
  Relational Operator1 : RelationalOperator  Operator===  OutDataTypeStr=boolean  RndMeth=Nearest
  Relational Operator2 : RelationalOperator  Operator===  OutDataTypeStr=boolean  RndMeth=Nearest
  Relational Operator3 : RelationalOperator  Operator===  OutDataTypeStr=boolean  RndMeth=Nearest
  StreamOut : Outport
  Ctrl : Outport  Port=2
  wires:
  Minus2/1 -> Relational Operator3/2, Relational Operator2/2
  Feature Row Counter/1 -> Relational Operator2/1, Relational Operator3/1, Compare To Zero/1
  Relational Operator2/1 -> Feature Row Counter/1
  Compare To Zero/1 -> Logical Operator/2
  Relational Operator3/1 -> Logical Operator2/1
  Feature_Area/1 -> Minus1/1
  Constant/1 -> Minus1/2
  Logical Operator/1 -> Logical Operator1/1
  Constant1/1 -> Minus2/2
  Feature_Width/1 -> Minus2/1
  Pixel Control Bus Creator/1 -> Ctrl/1
  Delay1/1 -> Feature Area Counter/2, Feature Row Counter/2, Logical Operator5/2, Logical Operator2/2, Logical Operator1/2, Logical Operator3/2, Pixel Control Bus Creator/5
  Delay36/1 -> StreamOut/1
  Logical Operator1/1 -> Pixel Control Bus Creator/1
  Logical Operator2/1 -> Pixel Control Bus Creator/2
  Logical Operator3/1 -> Pixel Control Bus Creator/4
  Logical Operator5/1 -> Pixel Control Bus Creator/3
  Feature Area Counter/1 -> Compare To Zero1/1, Relational Operator1/1
  Minus1/1 -> Relational Operator1/2
  Relational Operator1/1 -> Feature Area Counter/1, Logical Operator3/1
  Compare To Zero1/1 -> Logical Operator/1, Logical Operator5/1
  Stream_In/1 -> Delay36/1
  Stream_Valid/1 -> Delay1/1

== system external_memory_test/DUT/2DConvPE V1.2/LIne Buffer/Line Buffer/CtrlGen ==
  note: valid
  note: vEnd
  note: vStart
  note: hEnd
  note: hstart
  Stream_In : Inport
  Stream_Valid : Inport  Port=2
  Feature_Area : Inport  Port=3
  Feature_Width : Inport  Port=4
  Compare To Zero : simulink/Logic and Bit Operations/Compare To Zero  relop===  OutDataTypeStr=boolean
  Compare To Zero1 : simulink/Logic and Bit Operations/Compare To Zero  relop===  OutDataTypeStr=boolean
  Constant : Constant  OutDataTypeStr=uint32  SampleTime=-1
  Constant1 : Constant  OutDataTypeStr=uint32  SampleTime=-1
  Delay3 : Delay  DelayLength=1
  Delay35 : Delay  DelayLength=1
  Feature Area Counter : hdlsllib/Sources/HDL Counter  CountType=Free running  CountInit=0  CountStep=1  CountMax=2^15  CountFromType=Initial value  CountFrom=0  CountResetPort=on  CountLoadPort=off  CountEnbPort=on  CountDirPort=off  CountDataType=Unsigned  CountWordLen=32  CountFracLen=0  CountSampTime=1
  Feature Row Counter : hdlsllib/Sources/HDL Counter  CountType=Free running  CountInit=0  CountStep=1  CountMax=2^15  CountFromType=Initial value  CountFrom=0  CountResetPort=on  CountLoadPort=off  CountEnbPort=on  CountDirPort=off  CountDataType=Unsigned  CountWordLen=32  CountFracLen=0  CountSampTime=1
  Logical Operator : Logic  Operator=OR  AllPortsSameDT=off  OutDataTypeStr=boolean
  Logical Operator{1..3,5} (4 alike) : Logic  AllPortsSameDT=off  OutDataTypeStr=boolean
  Minus1 : Sum  Inputs=+-
  Minus2 : Sum  Inputs=+-
  Pixel Control Bus Creator : visionhdlutilities/Pixel Control Bus Creator
      settings: SourceProductBaseCode=VT
  Relational Operator1 : RelationalOperator  Operator===  OutDataTypeStr=boolean  RndMeth=Nearest
  Relational Operator2 : RelationalOperator  Operator===  OutDataTypeStr=boolean  RndMeth=Nearest
  Relational Operator3 : RelationalOperator  Operator===  OutDataTypeStr=boolean  RndMeth=Nearest
  StreamOut : Outport
  Ctrl : Outport  Port=2
  wires:
  Minus2/1 -> Relational Operator3/2, Relational Operator2/2
  Feature Row Counter/1 -> Relational Operator2/1, Relational Operator3/1, Compare To Zero/1
  Relational Operator2/1 -> Feature Row Counter/1
  Compare To Zero/1 -> Logical Operator/2
  Relational Operator3/1 -> Logical Operator2/1
  Feature_Area/1 -> Minus1/1
  Constant/1 -> Minus1/2
  Logical Operator/1 -> Logical Operator1/1
  Constant1/1 -> Minus2/2
  Feature_Width/1 -> Minus2/1
  Pixel Control Bus Creator/1 -> Ctrl/1
  Delay3/1 -> Feature Area Counter/2, Feature Row Counter/2, Logical Operator5/2, Logical Operator2/2, Logical Operator1/2, Logical Operator3/2, Pixel Control Bus Creator/5
  Stream_In/1 -> Delay35/1
  Logical Operator1/1 -> Pixel Control Bus Creator/1
  Logical Operator2/1 -> Pixel Control Bus Creator/2
  Logical Operator3/1 -> Pixel Control Bus Creator/4
  Logical Operator5/1 -> Pixel Control Bus Creator/3
  Feature Area Counter/1 -> Compare To Zero1/1, Relational Operator1/1
  Minus1/1 -> Relational Operator1/2
  Relational Operator1/1 -> Feature Area Counter/1, Logical Operator3/1
  Compare To Zero1/1 -> Logical Operator/1, Logical Operator5/1
  Delay35/1 -> StreamOut/1
  Stream_Valid/1 -> Delay3/1

== system external_memory_test/DUT/2DConvPE V1.2/MaxPooling/Line Buffer1/CtrlGen ==
  note: valid
  note: vEnd
  note: vStart
  note: hEnd
  note: hstart
  Stream_In : Inport
  Stream_Valid : Inport  Port=2
  Feature_Area : Inport  Port=3
  Feature_Width : Inport  Port=4
  Compare To Zero : simulink/Logic and Bit Operations/Compare To Zero  relop===  OutDataTypeStr=boolean
  Compare To Zero1 : simulink/Logic and Bit Operations/Compare To Zero  relop===  OutDataTypeStr=boolean
  Constant : Constant  OutDataTypeStr=uint32  SampleTime=-1
  Constant1 : Constant  OutDataTypeStr=uint32  SampleTime=-1
  Delay1 : Delay  DelayLength=1
  Delay36 : Delay  DelayLength=1
  Feature Area Counter : hdlsllib/Sources/HDL Counter  CountType=Free running  CountInit=0  CountStep=1  CountMax=2^15  CountFromType=Initial value  CountFrom=0  CountResetPort=on  CountLoadPort=off  CountEnbPort=on  CountDirPort=off  CountDataType=Unsigned  CountWordLen=32  CountFracLen=0  CountSampTime=1
  Feature Row Counter : hdlsllib/Sources/HDL Counter  CountType=Free running  CountInit=0  CountStep=1  CountMax=2^15  CountFromType=Initial value  CountFrom=0  CountResetPort=on  CountLoadPort=off  CountEnbPort=on  CountDirPort=off  CountDataType=Unsigned  CountWordLen=32  CountFracLen=0  CountSampTime=1
  Logical Operator : Logic  Operator=OR  AllPortsSameDT=off  OutDataTypeStr=boolean
  Logical Operator{1..3,5} (4 alike) : Logic  AllPortsSameDT=off  OutDataTypeStr=boolean
  Minus1 : Sum  Inputs=+-
  Minus2 : Sum  Inputs=+-
  Pixel Control Bus Creator : visionhdlutilities/Pixel Control Bus Creator
      settings: SourceProductBaseCode=VT
  Relational Operator1 : RelationalOperator  Operator===  OutDataTypeStr=boolean  RndMeth=Nearest
  Relational Operator2 : RelationalOperator  Operator===  OutDataTypeStr=boolean  RndMeth=Nearest
  Relational Operator3 : RelationalOperator  Operator===  OutDataTypeStr=boolean  RndMeth=Nearest
  StreamOut : Outport
  Ctrl : Outport  Port=2
  wires:
  Minus2/1 -> Relational Operator3/2, Relational Operator2/2
  Feature Row Counter/1 -> Relational Operator2/1, Relational Operator3/1, Compare To Zero/1
  Relational Operator2/1 -> Feature Row Counter/1
  Compare To Zero/1 -> Logical Operator/2
  Relational Operator3/1 -> Logical Operator2/1
  Feature_Area/1 -> Minus1/1
  Constant/1 -> Minus1/2
  Logical Operator/1 -> Logical Operator1/1
  Constant1/1 -> Minus2/2
  Feature_Width/1 -> Minus2/1
  Pixel Control Bus Creator/1 -> Ctrl/1
  Delay1/1 -> Feature Area Counter/2, Feature Row Counter/2, Logical Operator5/2, Logical Operator2/2, Logical Operator1/2, Logical Operator3/2, Pixel Control Bus Creator/5
  Delay36/1 -> StreamOut/1
  Logical Operator1/1 -> Pixel Control Bus Creator/1
  Logical Operator2/1 -> Pixel Control Bus Creator/2
  Logical Operator3/1 -> Pixel Control Bus Creator/4
  Logical Operator5/1 -> Pixel Control Bus Creator/3
  Feature Area Counter/1 -> Compare To Zero1/1, Relational Operator1/1
  Minus1/1 -> Relational Operator1/2
  Relational Operator1/1 -> Feature Area Counter/1, Logical Operator3/1
  Compare To Zero1/1 -> Logical Operator/1, Logical Operator5/1
  Stream_In/1 -> Delay36/1
  Stream_Valid/1 -> Delay1/1

== system external_memory_test/DUT/2DConvPE V1.3/LIne Buffer/Line Buffer/CtrlGen ==
  note: valid
  note: vEnd
  note: vStart
  note: hEnd
  note: hstart
  Stream_In : Inport
  Stream_Valid : Inport  Port=2
  Feature_Area : Inport  Port=3
  Feature_Width : Inport  Port=4
  Compare To Zero : simulink/Logic and Bit Operations/Compare To Zero  relop===  OutDataTypeStr=boolean
  Compare To Zero1 : simulink/Logic and Bit Operations/Compare To Zero  relop===  OutDataTypeStr=boolean
  Constant : Constant  OutDataTypeStr=uint32  SampleTime=-1
  Constant1 : Constant  OutDataTypeStr=uint32  SampleTime=-1
  Delay3 : Delay  DelayLength=1
  Delay35 : Delay  DelayLength=1
  Feature Area Counter : hdlsllib/Sources/HDL Counter  CountType=Free running  CountInit=0  CountStep=1  CountMax=2^15  CountFromType=Initial value  CountFrom=0  CountResetPort=on  CountLoadPort=off  CountEnbPort=on  CountDirPort=off  CountDataType=Unsigned  CountWordLen=32  CountFracLen=0  CountSampTime=1
  Feature Row Counter : hdlsllib/Sources/HDL Counter  CountType=Free running  CountInit=0  CountStep=1  CountMax=2^15  CountFromType=Initial value  CountFrom=0  CountResetPort=on  CountLoadPort=off  CountEnbPort=on  CountDirPort=off  CountDataType=Unsigned  CountWordLen=32  CountFracLen=0  CountSampTime=1
  Logical Operator : Logic  Operator=OR  AllPortsSameDT=off  OutDataTypeStr=boolean
  Logical Operator{1..3,5} (4 alike) : Logic  AllPortsSameDT=off  OutDataTypeStr=boolean
  Minus1 : Sum  Inputs=+-
  Minus2 : Sum  Inputs=+-
  Pixel Control Bus Creator : visionhdlutilities/Pixel Control Bus Creator
      settings: SourceProductBaseCode=VT
  Relational Operator1 : RelationalOperator  Operator===  OutDataTypeStr=boolean  RndMeth=Nearest
  Relational Operator2 : RelationalOperator  Operator===  OutDataTypeStr=boolean  RndMeth=Nearest
  Relational Operator3 : RelationalOperator  Operator===  OutDataTypeStr=boolean  RndMeth=Nearest
  StreamOut : Outport
  Ctrl : Outport  Port=2
  wires:
  Minus2/1 -> Relational Operator3/2, Relational Operator2/2
  Feature Row Counter/1 -> Relational Operator2/1, Relational Operator3/1, Compare To Zero/1
  Relational Operator2/1 -> Feature Row Counter/1
  Compare To Zero/1 -> Logical Operator/2
  Relational Operator3/1 -> Logical Operator2/1
  Feature_Area/1 -> Minus1/1
  Constant/1 -> Minus1/2
  Logical Operator/1 -> Logical Operator1/1
  Constant1/1 -> Minus2/2
  Feature_Width/1 -> Minus2/1
  Pixel Control Bus Creator/1 -> Ctrl/1
  Delay3/1 -> Feature Area Counter/2, Feature Row Counter/2, Logical Operator5/2, Logical Operator2/2, Logical Operator1/2, Logical Operator3/2, Pixel Control Bus Creator/5
  Stream_In/1 -> Delay35/1
  Logical Operator1/1 -> Pixel Control Bus Creator/1
  Logical Operator2/1 -> Pixel Control Bus Creator/2
  Logical Operator3/1 -> Pixel Control Bus Creator/4
  Logical Operator5/1 -> Pixel Control Bus Creator/3
  Feature Area Counter/1 -> Compare To Zero1/1, Relational Operator1/1
  Minus1/1 -> Relational Operator1/2
  Relational Operator1/1 -> Feature Area Counter/1, Logical Operator3/1
  Compare To Zero1/1 -> Logical Operator/1, Logical Operator5/1
  Delay35/1 -> StreamOut/1
  Stream_Valid/1 -> Delay3/1

== system external_memory_test/DUT/2DConvPE V1.3/MaxPooling/Line Buffer1/CtrlGen ==
  note: valid
  note: vEnd
  note: vStart
  note: hEnd
  note: hstart
  Stream_In : Inport
  Stream_Valid : Inport  Port=2
  Feature_Area : Inport  Port=3
  Feature_Width : Inport  Port=4
  Compare To Zero : simulink/Logic and Bit Operations/Compare To Zero  relop===  OutDataTypeStr=boolean
  Compare To Zero1 : simulink/Logic and Bit Operations/Compare To Zero  relop===  OutDataTypeStr=boolean
  Constant : Constant  OutDataTypeStr=uint32  SampleTime=-1
  Constant1 : Constant  OutDataTypeStr=uint32  SampleTime=-1
  Delay1 : Delay  DelayLength=1
  Delay36 : Delay  DelayLength=1
  Feature Area Counter : hdlsllib/Sources/HDL Counter  CountType=Free running  CountInit=0  CountStep=1  CountMax=2^15  CountFromType=Initial value  CountFrom=0  CountResetPort=on  CountLoadPort=off  CountEnbPort=on  CountDirPort=off  CountDataType=Unsigned  CountWordLen=32  CountFracLen=0  CountSampTime=1
  Feature Row Counter : hdlsllib/Sources/HDL Counter  CountType=Free running  CountInit=0  CountStep=1  CountMax=2^15  CountFromType=Initial value  CountFrom=0  CountResetPort=on  CountLoadPort=off  CountEnbPort=on  CountDirPort=off  CountDataType=Unsigned  CountWordLen=32  CountFracLen=0  CountSampTime=1
  Logical Operator : Logic  Operator=OR  AllPortsSameDT=off  OutDataTypeStr=boolean
  Logical Operator{1..3,5} (4 alike) : Logic  AllPortsSameDT=off  OutDataTypeStr=boolean
  Minus1 : Sum  Inputs=+-
  Minus2 : Sum  Inputs=+-
  Pixel Control Bus Creator : visionhdlutilities/Pixel Control Bus Creator
      settings: SourceProductBaseCode=VT
  Relational Operator1 : RelationalOperator  Operator===  OutDataTypeStr=boolean  RndMeth=Nearest
  Relational Operator2 : RelationalOperator  Operator===  OutDataTypeStr=boolean  RndMeth=Nearest
  Relational Operator3 : RelationalOperator  Operator===  OutDataTypeStr=boolean  RndMeth=Nearest
  StreamOut : Outport
  Ctrl : Outport  Port=2
  wires:
  Minus2/1 -> Relational Operator3/2, Relational Operator2/2
  Feature Row Counter/1 -> Relational Operator2/1, Relational Operator3/1, Compare To Zero/1
  Relational Operator2/1 -> Feature Row Counter/1
  Compare To Zero/1 -> Logical Operator/2
  Relational Operator3/1 -> Logical Operator2/1
  Feature_Area/1 -> Minus1/1
  Constant/1 -> Minus1/2
  Logical Operator/1 -> Logical Operator1/1
  Constant1/1 -> Minus2/2
  Feature_Width/1 -> Minus2/1
  Pixel Control Bus Creator/1 -> Ctrl/1
  Delay1/1 -> Feature Area Counter/2, Feature Row Counter/2, Logical Operator5/2, Logical Operator2/2, Logical Operator1/2, Logical Operator3/2, Pixel Control Bus Creator/5
  Delay36/1 -> StreamOut/1
  Logical Operator1/1 -> Pixel Control Bus Creator/1
  Logical Operator2/1 -> Pixel Control Bus Creator/2
  Logical Operator3/1 -> Pixel Control Bus Creator/4
  Logical Operator5/1 -> Pixel Control Bus Creator/3
  Feature Area Counter/1 -> Compare To Zero1/1, Relational Operator1/1
  Minus1/1 -> Relational Operator1/2
  Relational Operator1/1 -> Feature Area Counter/1, Logical Operator3/1
  Compare To Zero1/1 -> Logical Operator/1, Logical Operator5/1
  Stream_In/1 -> Delay36/1
  Stream_Valid/1 -> Delay1/1

== matlab function external_memory_test/DUT/2DConvPE V1.1/MATLAB Function ==
  settings: fimath=fimath('RoundingMethod', 'Floor','OverflowAction', 'Wrap','ProductMode', 'FullPrecision', 'SumMode', 'FullPrecision')
  data: w0 output; dataIn input; w1 output; rst input; write_en input; w2 output; w3 output; w4 output; w5 output; w6 output; w7 output; w8 output
function [w0, w1, w2, w3 , w4, w5, w6, w7, w8] = weight_register(dataIn, rst, write_en)
%#codegen
persistent read_cnt;

% Counter
if(isempty(read_cnt))
   read_cnt = fi(0,1,32,0); 
end

% Max Count = uint32(8)
persistent cntMax;

if(isempty(cntMax))
   cntMax = fi(9 - 1,1,32,0);
end

% weight0
persistent weight0
if(isempty(weight0))
   weight0 = fi(0,1,32,0); 
end

% weight1
persistent weight1
if(isempty(weight1))
   weight1 = fi(0,1,32,0); 
end

% weight2
persistent weight2
if(isempty(weight2))
   weight2 = fi(0,1,32,0); 
end

% weight3
persistent weight3
if(isempty(weight3))
   weight3 = fi(0,1,32,0); 
end

% weight1
persistent weight4
if(isempty(weight4))
   weight4 = fi(0,1,32,0); 
end

% weight5
persistent weight5
if(isempty(weight5))
   weight5 = fi(0,1,32,0); 
end

% weight6
persistent weight6
if(isempty(weight6))
   weight6 = fi(0,1,32,0); 
end

% weight7
persistent weight7
if(isempty(weight7))
   weight7 = fi(0,1,32,0); 
end

% weight8
persistent weight8
if(isempty(weight8))
   weight8 = fi(0,1,32,0); 
end

%%%%%%%%%%%%%%%%%%%%%%%%%%%%%%%%%%%%
% Output Logic
    w0 = weight0;
    w1 = weight1;
    w2 = weight2;
    w3 = weight3;
    w4 = weight4;
    w5 = weight5;
    w6 = weight6;
    w7 = weight7;
    w8 = weight8;
%%%%%%%%%%%%%%%%%%%%%%%%%%%%%%%%%%%%

if (rst == 1)
    % reset the output
    read_cnt = fi(0,1,32,0);
    
    weight0 = fi(0,1,32,0);
    weight1 = fi(0,1,32,0);
    weight2 = fi(0,1,32,0);
    weight3 = fi(0,1,32,0);
    weight4 = fi(0,1,32,0);
    weight5 = fi(0,1,32,0);
    weight6 = fi(0,1,32,0);
    weight7 = fi(0,1,32,0);
    weight8 = fi(0,1,32,0);
elseif (write_en == 1)
    if (read_cnt == cntMax)
        read_cnt = fi(0,1,32,0);
        weight0 = fi(dataIn,1,32,0);
    else
        if (read_cnt == 0)
           weight8 = fi(dataIn,1,32,0);
        elseif (read_cnt == 1)
            weight5 = fi(dataIn,1,32,0);
        elseif (read_cnt == 2)
            weight2 = fi(dataIn,1,32,0);
        elseif (read_cnt == 3)
            weight7 = fi(dataIn,1,32,0);
        elseif (read_cnt == 4)
            weight4 = fi(dataIn,1,32,0);
        elseif (read_cnt == 5)
            weight1 = fi(dataIn,1,32,0);
        elseif (read_cnt == 6)
            weight6 = fi(dataIn,1,32,0);
        elseif (read_cnt == 7)
            weight3 = fi(dataIn,1,32,0);
        end   
        read_cnt = fi(read_cnt+1, 1,32,0);
    end
end
